simulink model "fig913"  (R2017a)
settings: Solver=FixedStepDiscrete  StartTime=0.0  StopTime=runtime  FixedStep=0.1  RelTol=1e-3  EnableMultiTasking=on
values from neighbouring files (symbols this model uses):
  e = 5    [test_round.m]    (also in test_straight.m = 10)
settings Model: Creator=a01209720  LastModifiedBy=a01209720
settings SolverCC: AutoInsertRateTranBlk=on
settings DataIOCC: LimitDataPoints=on
settings OptimizationCC: LifeSpan=inf
settings DebuggingCC: AllowSymbolicDim=off  SFUnexpectedBacktrackingDiag=warning  SFNoUnconditionalDefaultTransitionDiag=warning  SFExecutionAtInitializationDiag=none
settings GRTTargetCC: TargetLangStandard=C89/C90 (ANSI)
settings ConfigComp: CovMetricSettings=dw  CovHtmlReporting=on  CovSaveCumulativeToWorkspaceVar=on  CovSaveSingleToWorkspaceVar=on  CovShowResultsExplorer=off  CovExternalEMLEnable=off

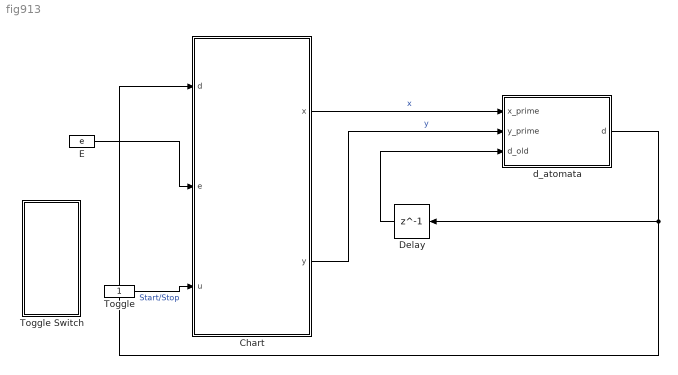
== system fig913 ==
  Chart : Stateflow chart  TreatAsAtomicUnit=on
  Delay : Delay  DelayLength=1  InitialCondition=0
  E : Constant  Value=e
  Toggle : Constant
  Toggle Switch : Subsystem  DialogController=hmiCreateDDGDialog  IsWebBlock=on  mask(MWDashboardBlock){webBlockId=9ce7b99b-8eaf-4cd0-9f7a-8e2d2923029e, webBlockType=toggleswitch, ShowInLibBrowser=on, ShowInitialText=on, HMISrcModelName=fig913}
      mask prompts: webBlockId "WebBlock Id"; webBlockType "WebBlock Type"; HMISrcModelName "Source Model"
      mask help: SimulinkHMI:dialogs:SwitchDialogDesc
      mask Help: helpview([docroot '/mapfiles/simulink.map'], 'hmi_toggle_switch')
      mask Display:
      | if strcmp(get_param(bdroot(gcb),'BlockDiagramType'), 'library')
      |     image([(matlabroot) '/toolbox/simulink/hmi/icons/ToggleSwitch.png']);
      | end
  d_atomata : MATLAB Function  TreatAsAtomicUnit=on
  wires:
  E/1 -> Chart/2(e)
  Chart/1(x) -> d_atomata/1(x_prime)  "x"
  Toggle/1 -> Chart/3(u)  "Start/Stop"
  Chart/2(y) -> d_atomata/2(y_prime)  "y"
  d_atomata/1(d) -> Delay/1, Chart/1(d)
  Delay/1 -> d_atomata/3(d_old)

== system fig913/Toggle Switch ==

== matlab function fig913/d_atomata ==
  data: x_prime input; d output; y_prime input; d_old input
function d = fcn(x_prime,y_prime,d_old)
  d = d_old+y_prime;

== stateflow chart fig913/Chart ==
  settings: stateMachineType=MOORE_MACHINE
  state Right %State Name
    x = ((v*cos(dir))/2)*dt; % entry action
    y = ((v*sin(dir))/2)*dt; % entry action
    dir =dir - pi*dt;
    %d >= e
    % during:
  state Straight
    x = (v*cos(dir))*dt; % entry action
    y = (v*sin(dir))*dt; % entry action
    dir = dir + 0;
    %-e <= d <= e
  state Stop
    x = 0; %x0;
    y = 0; %y0;
    dir = dir + 0; %theta0;
  state Left
    x = ((v*cos(dir))/2)*dt; % entry action
    y = ((v*sin(dir))/2)*dt; % entry action
    dir = dir + pi*dt;
  Right %State Name -> Right %State Name [order 3]
  Straight -> Straight [order 4] : [-e <= d <= e]
  Right %State Name -> Straight [order 1] : [d <= e]
      | % [transition condition]{action}
  Straight -> Right %State Name [order 1] : [d >= e]
  Straight -> Stop [order 2] : [u == 0]
  Stop -> Straight [order 2] : [u == 1 & -e <= d <= e]
  Straight -> Left [order 3] : [d <= -e]
  Left -> Straight [order 1] : [d >= -e]
  Right %State Name -> Stop [order 2] : [u == 0]
  Stop -> Right %State Name [order 1] : [u == 1 & d >= e]
  (default) -> Stop
  Left -> Stop [order 2] : [u == 0]
  Stop -> Left [order 3] : [u == 1 & d <= -e]
  Stop -> Stop [order 4]
  Left -> Left [order 3] : [d <= -e]
  data: x output =x0; y output =y0; d input; e input; u input; dir local double =theta0; v constant double =v; dt constant double =dt
